simulink model "T1_NonLinear_2_dof_Helicopter"  (R2023a)
settings: Solver=ode4  StartTime=0.0  StopTime=inf  FixedStep=0.1  RelTol=1e-3
values from neighbouring files (symbols this model uses):
  B_p = 0.01    [Heli_Parameters.m]
  B_y = 0.08    [Heli_Parameters.m]
  g = 9.81    [Heli_Parameters.m]
  J_eqp = 0.0172    [Heli_Parameters.m]
  J_eqy = 0.0210    (= 0.021)    [Heli_Parameters.m]
  K_pp = 0.0556    [Heli_Parameters.m]
  K_py = 0.005    [Heli_Parameters.m]
  K_yp = 0.15    [Heli_Parameters.m]
  K_yy = 0.21084    [Heli_Parameters.m]
  l_cm = 0.015    [Heli_Parameters.m]
  m_heli = 0.479    [Heli_Parameters.m]
libraries: realtime_pacer_lib x1
settings Model: Creator=aleho  LastModifiedBy=aleho

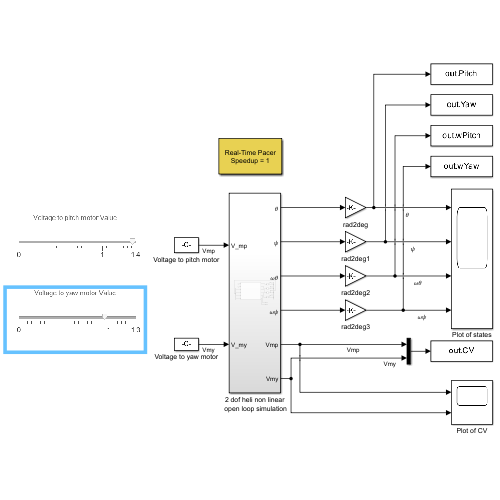
[thumbnail: Simulink's stored preview of the top-level diagram]
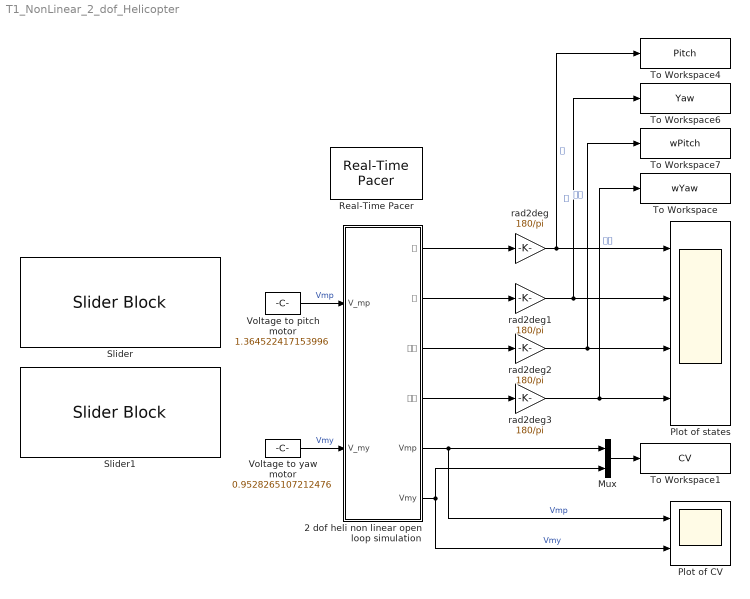
== system T1_NonLinear_2_dof_Helicopter ==
  2 dof heli non linear open loop simulation : Subsystem
  Mux : Mux  Inputs=2
  Plot of CV : Scope  NumInputPorts=2
  Plot of states : Scope  NumInputPorts=4
  Real-Time Pacer : realtime_pacer_lib/Real-Time Pacer  simTimePerRealTime=1
      settings: SourceProductName=Real-Time Pacer
  Slider : SliderBlock  ScaleMax=1.4  TickInterval=1
  Slider1 : SliderBlock  ScaleMax=1.3  TickInterval=1
  To Workspace : ToWorkspace  VariableName=wYaw  SaveFormat=Timeseries  SampleTime=-1
  To Workspace1 : ToWorkspace  VariableName=CV  SaveFormat=Timeseries  SampleTime=-1
  To Workspace4 : ToWorkspace  VariableName=Pitch  SaveFormat=Timeseries  SampleTime=-1
  To Workspace6 : ToWorkspace  VariableName=Yaw  SaveFormat=Timeseries  SampleTime=-1
  To Workspace7 : ToWorkspace  VariableName=wPitch  SaveFormat=Timeseries  SampleTime=-1
  Voltage to pitch motor : Constant  Value=1.364522417153996
  Voltage to yaw motor : Constant  Value=0.9528265107212476
  rad2deg{,1..3} (4 alike) : Gain  Gain=180/pi
  wires:
  rad2deg2/1 -> To Workspace7/1, Plot of states/3  "𝜔𝜃"
  rad2deg3/1 -> To Workspace/1, Plot of states/4  "𝜔𝜓"
  Voltage to pitch motor/1 -> 2 dof heli non linear open loop simulation/1(V_mp)  "Vmp"
  Voltage to yaw motor/1 -> 2 dof heli non linear open loop simulation/2(V_my)  "Vmy"
  2 dof heli non linear open loop simulation/1(𝜃) -> rad2deg/1
  2 dof heli non linear open loop simulation/2(𝜓) -> rad2deg1/1
  2 dof heli non linear open loop simulation/3(𝜔𝜃) -> rad2deg2/1
  2 dof heli non linear open loop simulation/4(𝜔𝜓) -> rad2deg3/1
  rad2deg/1 -> To Workspace4/1, Plot of states/1  "𝜃"
  rad2deg1/1 -> To Workspace6/1, Plot of states/2  "𝜓"
  2 dof heli non linear open loop simulation/5(Vmp) -> Plot of CV/1, Mux/1  "Vmp"
  2 dof heli non linear open loop simulation/6(Vmy) -> Mux/2, Plot of CV/2  "Vmy"
  Mux/1 -> To Workspace1/1

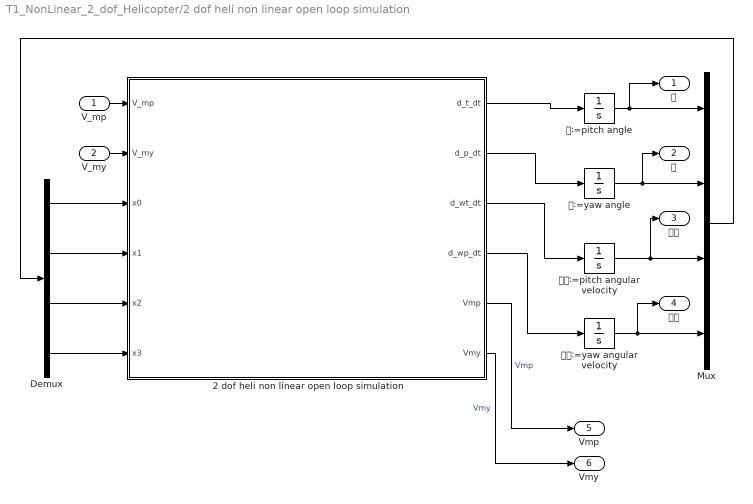
== system T1_NonLinear_2_dof_Helicopter/2 dof heli non linear open loop simulation ==
  V_mp : Inport
  V_my : Inport  Port=2
  2 dof heli non linear open loop simulation : MATLAB Function  TreatAsAtomicUnit=on
  Demux : Demux
  Mux : Mux
  𝜃∶=pitch angle : Integrator  InitialCondition=-45*pi/180  LimitOutput=on  UpperSaturationLimit=pi/4  LowerSaturationLimit=-pi/4
  𝜓∶=yaw angle : Integrator  InitialCondition=pi/2  LimitOutput=on  UpperSaturationLimit=pi  LowerSaturationLimit=0
  𝜔𝜃∶=pitch angular velocity : Integrator
  𝜔𝜓∶=yaw angular velocity : Integrator
  𝜃 : Outport
  𝜓 : Outport  Port=2
  𝜔𝜃 : Outport  Port=3
  𝜔𝜓 : Outport  Port=4
  Vmp : Outport  Port=5
  Vmy : Outport  Port=6
  wires:
  V_mp/1 -> 2 dof heli non linear open loop simulation/1(V_mp)
  𝜔𝜃∶=pitch angular velocity/1 -> 𝜔𝜃/1, Mux/3
  Demux/4 -> 2 dof heli non linear open loop simulation/6(x3)
  𝜔𝜓∶=yaw angular velocity/1 -> 𝜔𝜓/1, Mux/4
  Mux/1 -> Demux/1
  𝜃∶=pitch angle/1 -> 𝜃/1, Mux/1
  𝜓∶=yaw angle/1 -> 𝜓/1, Mux/2
  2 dof heli non linear open loop simulation/1(d_t_dt) -> 𝜃∶=pitch angle/1
  V_my/1 -> 2 dof heli non linear open loop simulation/2(V_my)
  Demux/1 -> 2 dof heli non linear open loop simulation/3(x0)
  Demux/3 -> 2 dof heli non linear open loop simulation/5(x2)
  Demux/2 -> 2 dof heli non linear open loop simulation/4(x1)
  2 dof heli non linear open loop simulation/2(d_p_dt) -> 𝜓∶=yaw angle/1
  2 dof heli non linear open loop simulation/4(d_wp_dt) -> 𝜔𝜓∶=yaw angular velocity/1
  2 dof heli non linear open loop simulation/3(d_wt_dt) -> 𝜔𝜃∶=pitch angular velocity/1
  2 dof heli non linear open loop simulation/5(Vmp) -> Vmp/1  "Vmp"
  2 dof heli non linear open loop simulation/6(Vmy) -> Vmy/1  "Vmy"

== matlab function T1_NonLinear_2_dof_Helicopter/2 dof heli non linear open loop simulation/2 dof heli non linear open loop simulation ==
  data: V_mp input; V_my input; d_t_dt output; d_p_dt output; d_wt_dt output; d_wp_dt output; x0 input; x1 input; x2 input; x3 input; l_cm parameter; m_heli parameter; J_eqp parameter; J_eqy parameter; g parameter; K_pp parameter; K_yy parameter; K_py parameter; K_yp parameter; B_p parameter; B_y parameter; Vmp output; Vmy output
function [d_t_dt,d_p_dt,d_wt_dt,d_wp_dt, Vmp,Vmy] =  heli_2_dof_ODE_eqs(V_mp,V_my,x0,x1,x2,x3,l_cm, m_heli, J_eqp, J_eqy, g, K_pp, K_yy, K_py, K_yp, B_p, B_y)
% States
t = x0;    % pitch angle ( theta )
p = x1;    % yaw angle ( psi )
wt = x2;   % pitch angular velocity ( Omega theta )
wp = x3;   % yaw angular velocity ( Omega psi )

% Control voltages
Vmp = V_mp;
Vmy = V_my;

% ODEs
% pitch angle
d_t_dt = wt;

% yaw angle
d_p_dt = wp;

% pitch angular velocity
d_wt_dt = ((K_pp*V_mp)/(J_eqp+m_heli*l_cm^2)) - ((K_py*V_my)/(J_eqp+m_heli*l_cm^2))...
    - ((B_p*wt+m_heli*wp^2*sin(t)*l_cm^2*cos(t)+m_heli*g*cos(t)*l_cm) / (J_eqp+m_heli*l_cm^2));

% yaw angular velocity
d_wp_dt = ((K_yp*V_mp)/(J_eqy+m_heli*cos(t)^2*l_cm^2)) -...
    ((K_yy*V_my)/(J_eqy+m_heli*cos(t)^2*l_cm^2)) +...
    ((2*m_heli*wp*sin(t)*l_cm^2*cos(t)*wt)/(J_eqy+m_heli*cos(t)^2*l_cm^2))...
    - ((B_y*wp)/(J_eqy+m_heli*cos(t)^2*l_cm^2));
